simulink model "Powertrain_Model"  (R2020a)
settings: Solver=VariableStepAuto  StartTime=0.0  StopTime=2474  RelTol=1e-3
undefined symbols (not defined in the file): Af, Bv, Cd, Crf, gear_ratio, mass, r, range, rho, slope_angle
libraries: autolibshared x1
settings Model: Creator=lenovo  LastModifiedBy=lenovo

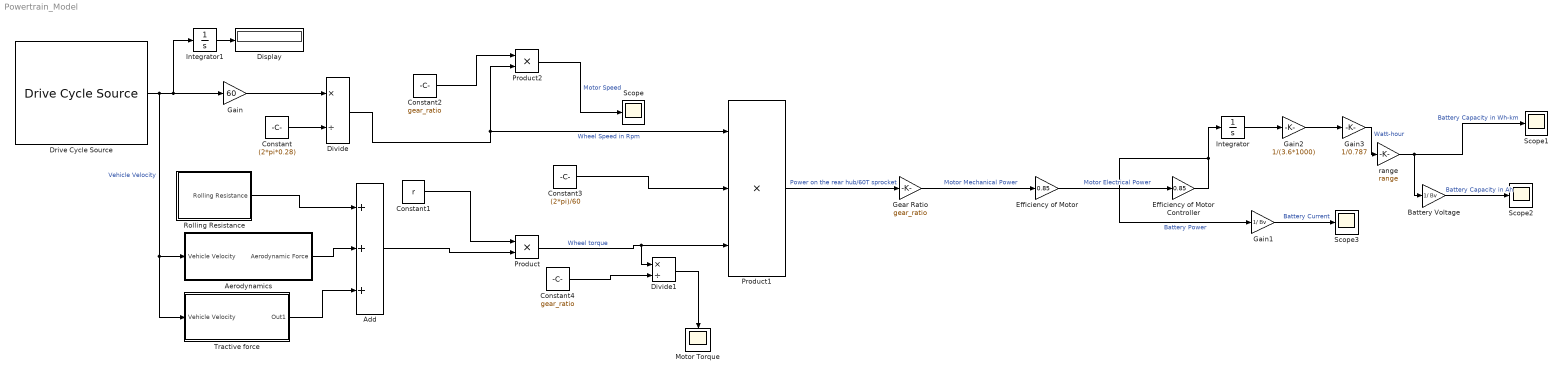
== system Powertrain_Model ==
  Add : Sum  Inputs=3
  Aerodynamics : Subsystem
  Battery Voltage : Gain  Gain=1/ Bv
  Constant : Constant  Value=(2*pi*0.28)
  Constant1 : Constant  Value=r
  Constant2 : Constant  Value=gear_ratio
  Constant3 : Constant  Value=(2*pi)/60
  Constant4 : Constant  Value=gear_ratio
  Display : Display
  Divide : Product  Inputs=*/
  Divide1 : Product  Inputs=*/
  Drive Cycle Source : autolibshared/Drive Cycle Source  cycleVar=FTP75  fileVar=cycleFTP75.mat  tfinal="2474  seconds"  cycleRepeat=off  outAccPort=off  outGearPort=off  gearList=No gear data  t_wot1=5  xdot_woto=0  xdot_wot1=30  t_wot2=20  xdot_wot2=0  t_wotend=30  srcUnit=m/s  outUnit=m/s  srcAccUnit=m/s/s  outAccUnit=m/s^2  dt=0  aMode=1  faultOption=off  velBnd=2  velBndUnit=mph  inUnit=m/s  timeBnd=1  failOption=off  stopSim=off  maxFaultCnt=10  maxFaultTime=2  maxTotFaultTime=15  traceOption=off  dtTrace=1  traceWindow=10  lastDCname=FTP75 Velocity  lastOutUnit=mph  lastDT=0  lastTB=1  lastSB=2  forceCalcBound=off
      settings: SourceProductBaseCode=PW,MT,VE,VP
  Efficiency of Motor : Gain  Gain=0.85
  Efficiency of Motor Controller : Gain  Gain=0.85
  Gain : Gain  Gain=60
  Gain1 : Gain  Gain=1/ Bv
  Gain2 : Gain  Gain=1/(3.6*1000)
  Gain3 : Gain  Gain=1/0.787
  Gear Ratio : Gain  Gain=gear_ratio
  Integrator : Integrator
  Integrator1 : Integrator
  Motor Torque : Scope
  Product : Product
  Product1 : Product  Inputs=3
  Product2 : Product
  Rolling Resistance : Subsystem
  Scope{,1..3} (4 alike) : Scope
  Tractive force : Subsystem
  range : Gain  Gain=range
  wires:
  Drive Cycle Source/1 -> Tractive force/1(Vehicle Velocity), Aerodynamics/1(Vehicle Velocity), Integrator1/1, Gain/1  "Vehicle Velocity"
  Gain/1 -> Divide/1
  Constant/1 -> Divide/2
  Divide/1 -> Product2/2, Product1/1  "Wheel Speed in Rpm"
  Rolling Resistance/1(Rolling Resistance) -> Add/1
  Aerodynamics/1(Aerodynamic Force) -> Add/2
  Tractive force/1(Out1) -> Add/3
  Constant1/1 -> Product/1
  Add/1 -> Product/2
  Product/1 -> Divide1/1, Product1/3  "Wheel torque"
  Product1/1 -> Gear Ratio/1  "Power on the rear hub/60T sprocket"
  Gear Ratio/1 -> Efficiency of Motor/1  "Motor Mechanical Power"
  Efficiency of Motor/1 -> Efficiency of Motor Controller/1  "Motor Electrical Power"
  Product2/1 -> Scope/1  "Motor Speed"
  Constant2/1 -> Product2/1
  Constant3/1 -> Product1/2
  Constant4/1 -> Divide1/2
  Divide1/1 -> Motor Torque/1
  Efficiency of Motor Controller/1 -> Gain1/1, Integrator/1  "Battery Power"
  Gain1/1 -> Scope3/1  "Battery Current"
  Integrator/1 -> Gain2/1
  Gain2/1 -> Gain3/1
  Gain3/1 -> range/1  "Watt-hour"
  range/1 -> Battery Voltage/1, Scope1/1  "Battery Capacity in Wh-km"
  Battery Voltage/1 -> Scope2/1  "Battery Capacity in Ah"
  Integrator1/1 -> Display/1

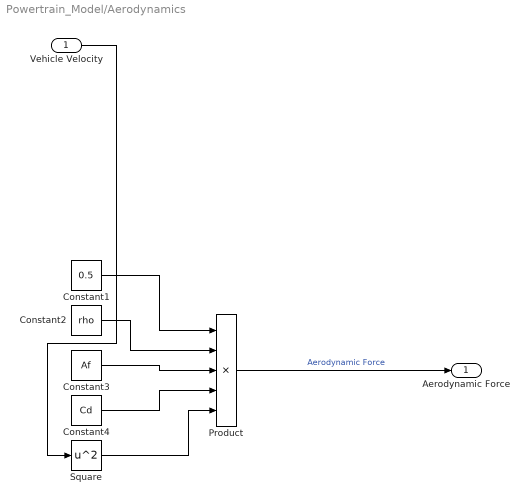
== system Powertrain_Model/Aerodynamics ==
  Vehicle Velocity : Inport
  Constant1 : Constant  Value=0.5
  Constant2 : Constant  Value=rho
  Constant3 : Constant  Value=Af
  Constant4 : Constant  Value=Cd
  Product : Product  Inputs=5
  Square : Math  Operator=square  SaturateOnIntegerOverflow=on
  Aerodynamic Force : Outport
  wires:
  Constant2/1 -> Product/2
  Constant3/1 -> Product/3
  Square/1 -> Product/5
  Constant1/1 -> Product/1
  Product/1 -> Aerodynamic Force/1  "Aerodynamic Force"
  Constant4/1 -> Product/4
  Vehicle Velocity/1 -> Square/1

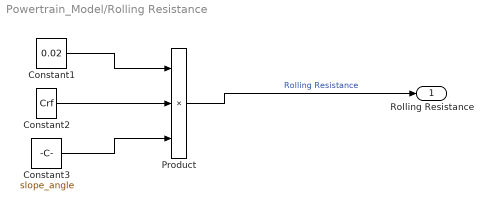
== system Powertrain_Model/Rolling Resistance ==
  Constant1 : Constant  Value=0.02
  Constant2 : Constant  Value=Crf
  Constant3 : Constant  Value=slope_angle
  Product : Product  Inputs=3
  Rolling Resistance : Outport
  wires:
  Constant2/1 -> Product/2
  Product/1 -> Rolling Resistance/1  "Rolling Resistance"
  Constant1/1 -> Product/1
  Constant3/1 -> Product/3

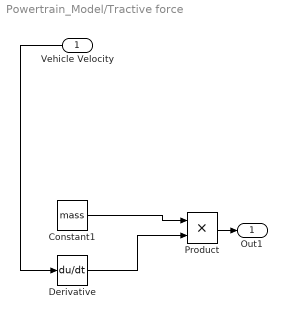
== system Powertrain_Model/Tractive force ==
  Vehicle Velocity : Inport
  Constant1 : Constant  Value=mass
  Derivative : Derivative
  Product : Product
  Out1 : Outport
  wires:
  Vehicle Velocity/1 -> Derivative/1
  Constant1/1 -> Product/1
  Product/1 -> Out1/1
  Derivative/1 -> Product/2
